simulink model "TASK8_trajectory_tracking"  (R2023b)
settings: Solver=VariableStepAuto  StartTime=0.0  StopTime=80  MaxStep=0.01  RelTol=1e-3  EnableMultiTasking=on
values from neighbouring files (symbols this model uses):
  b = 0.2    [TASK0_main_code.m]
  g = 9.81    [TASK0_main_code.m]
  J_s = 1/3*m*l^2    (= 4.99725166667)    [TASK0_main_code.m]
  K = place(A_lin, B_lin, p)    [TASK0_main_code.m]
  K1 = place(A_lin, B_lin, p1)    [TASK0_main_code.m]
  K2 = place(A_lin, B_lin, p2)    [TASK0_main_code.m]
  K3 = place(A_lin, B_lin, p3)    [TASK0_main_code.m]
  l = 3.11    [TASK0_main_code.m]
  m = 1.55    [TASK0_main_code.m]
  M = 7.87    [TASK0_main_code.m]
  N = [0; 0; 1; 0]    [TASK0_main_code.m]
libraries: dspinverses x4
settings Model: Creator=iklod_000  LastModifiedBy=piri
settings SolverCC: AlgebraicLoopSolver=TrustRegion
settings DataIOCC: ReturnWorkspaceOutputs=off
settings OptimizationCC: LifeSpan=inf
settings DebuggingCC: UnconnectedInputMsg=warning  UnconnectedOutputMsg=warning  UnconnectedLineMsg=warning  SFUnexpectedBacktrackingDiag=warning  SFNoUnconditionalDefaultTransitionDiag=warning  ArithmeticOperatorsInVariantConditions=warning
settings ModelReferenceCC: EnableRefExpFcnMdlSchedulingChecks=on
settings SFSimCC: SimUseLocalCustomCode=off  CustomCodeUndefinedFunction=UseInterfaceOnly
settings RTWCC: RTWUseLocalCustomCode=off
settings CodeAppCC: StateflowObjectComments=on
settings GRTTargetCC: TargetLangStandard=C89/C90 (ANSI)
settings ConfigComp: CovMetricSettings=dw  CovSaveCumulativeToWorkspaceVar=on  CovSaveSingleToWorkspaceVar=on  CovExternalEMLEnable=off

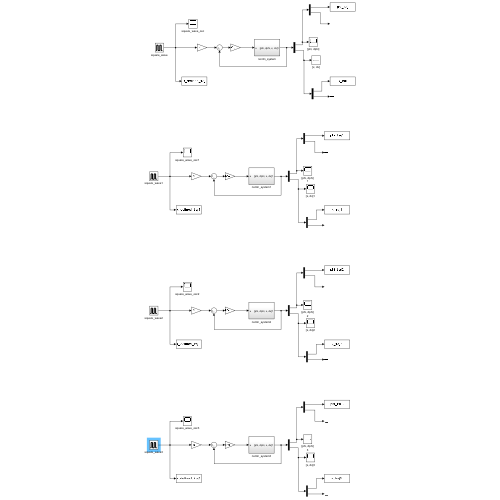
[thumbnail: Simulink's stored preview of the top-level diagram]
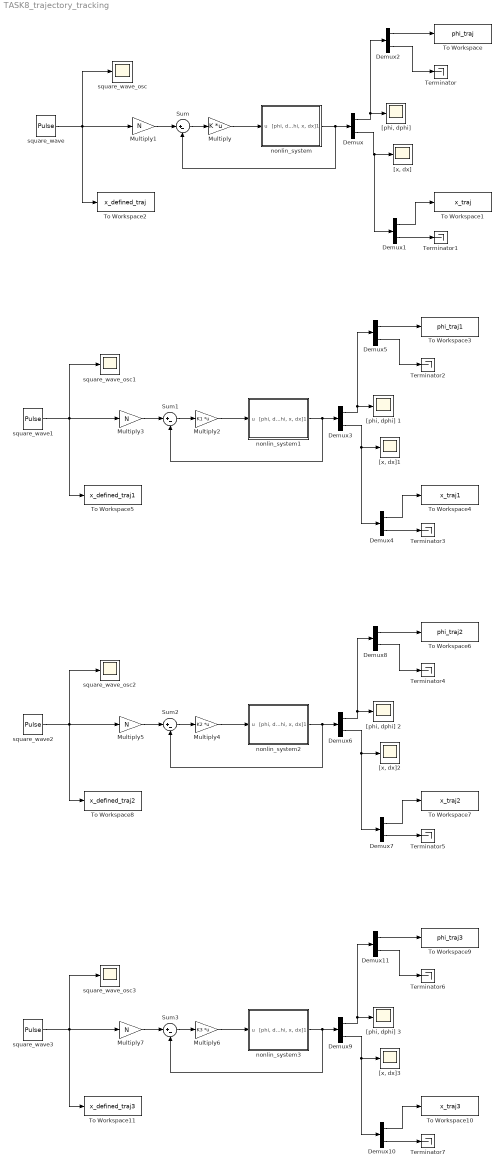
== system TASK8_trajectory_tracking ==
  Demux{,1..11} (12 alike) : Demux  Outputs=2
  Multiply : Gain  Gain=K  Multiplication=Matrix(K*u)
  Multiply{1,3,5,7} (4 alike) : Gain  Gain=N
  Multiply2 : Gain  Gain=K1  Multiplication=Matrix(K*u)
  Multiply4 : Gain  Gain=K2  Multiplication=Matrix(K*u)
  Multiply6 : Gain  Gain=K3  Multiplication=Matrix(K*u)
  Sum{,1..3} (4 alike) : Sum  Inputs=|+-
  Terminator{,1..7} (8 alike) : Terminator
  To Workspace : ToWorkspace  VariableName=phi_traj  SaveFormat=Timeseries  SampleTime=-1
  To Workspace1 : ToWorkspace  VariableName=x_traj  SaveFormat=Timeseries  SampleTime=-1
  To Workspace10 : ToWorkspace  VariableName=x_traj3  SaveFormat=Timeseries  SampleTime=-1
  To Workspace11 : ToWorkspace  VariableName=x_defined_traj3  SaveFormat=Timeseries  SampleTime=-1
  To Workspace2 : ToWorkspace  VariableName=x_defined_traj  SaveFormat=Timeseries  SampleTime=-1
  To Workspace3 : ToWorkspace  VariableName=phi_traj1  SaveFormat=Timeseries  SampleTime=-1
  To Workspace4 : ToWorkspace  VariableName=x_traj1  SaveFormat=Timeseries  SampleTime=-1
  To Workspace5 : ToWorkspace  VariableName=x_defined_traj1  SaveFormat=Timeseries  SampleTime=-1
  To Workspace6 : ToWorkspace  VariableName=phi_traj2  SaveFormat=Timeseries  SampleTime=-1
  To Workspace7 : ToWorkspace  VariableName=x_traj2  SaveFormat=Timeseries  SampleTime=-1
  To Workspace8 : ToWorkspace  VariableName=x_defined_traj2  SaveFormat=Timeseries  SampleTime=-1
  To Workspace9 : ToWorkspace  VariableName=phi_traj3  SaveFormat=Timeseries  SampleTime=-1
  [phi, dphi] {,1..3} (4 alike) : Scope
  [x, dx]{,1..3} (4 alike) : Scope
  nonlin_system : Subsystem
  nonlin_system1 : Subsystem
  nonlin_system2 : Subsystem
  nonlin_system3 : Subsystem
  square_wave{,1..3} (4 alike) : DiscretePulseGenerator  PulseType=Time based  Period=30  PulseWidth=50  PhaseDelay=15
  square_wave_osc{,1..3} (4 alike) : Scope
  wires:
  nonlin_system/1("[phi, dphi, x, dx]1") -> Sum/2, Demux/1
  Demux/1 -> Demux2/1, "[phi, dphi] "/1
  Demux/2 -> Demux1/1, "[x, dx]"/1
  Demux1/2 -> Terminator1/1
  Demux1/1 -> To Workspace1/1
  Demux2/1 -> To Workspace/1
  Demux2/2 -> Terminator/1
  Multiply/1 -> nonlin_system/1(u)
  Sum/1 -> Multiply/1
  Multiply1/1 -> Sum/1
  square_wave/1 -> square_wave_osc/1, To Workspace2/1, Multiply1/1
  Multiply3/1 -> Sum1/1
  Multiply2/1 -> nonlin_system1/1(u)
  square_wave1/1 -> square_wave_osc1/1, To Workspace5/1, Multiply3/1
  Demux3/1 -> Demux5/1, "[phi, dphi] 1"/1
  Demux5/1 -> To Workspace3/1
  Demux5/2 -> Terminator2/1
  Demux4/2 -> Terminator3/1
  nonlin_system1/1("[phi, dphi, x, dx]1") -> Sum1/2, Demux3/1
  Demux4/1 -> To Workspace4/1
  Demux3/2 -> Demux4/1, "[x, dx]1"/1
  Sum1/1 -> Multiply2/1
  Demux7/1 -> To Workspace7/1
  Demux6/2 -> Demux7/1, "[x, dx]2"/1
  Sum2/1 -> Multiply4/1
  Multiply4/1 -> nonlin_system2/1(u)
  Multiply5/1 -> Sum2/1
  square_wave2/1 -> square_wave_osc2/1, To Workspace8/1, Multiply5/1
  nonlin_system2/1("[phi, dphi, x, dx]1") -> Sum2/2, Demux6/1
  Demux8/2 -> Terminator4/1
  Demux8/1 -> To Workspace6/1
  Demux7/2 -> Terminator5/1
  Demux6/1 -> Demux8/1, "[phi, dphi] 2"/1
  Demux10/1 -> To Workspace10/1
  Demux9/2 -> Demux10/1, "[x, dx]3"/1
  Sum3/1 -> Multiply6/1
  Multiply6/1 -> nonlin_system3/1(u)
  Multiply7/1 -> Sum3/1
  square_wave3/1 -> square_wave_osc3/1, To Workspace11/1, Multiply7/1
  nonlin_system3/1("[phi, dphi, x, dx]1") -> Sum3/2, Demux9/1
  Demux11/2 -> Terminator6/1
  Demux11/1 -> To Workspace9/1
  Demux10/2 -> Terminator7/1
  Demux9/1 -> Demux11/1, "[phi, dphi] 3"/1

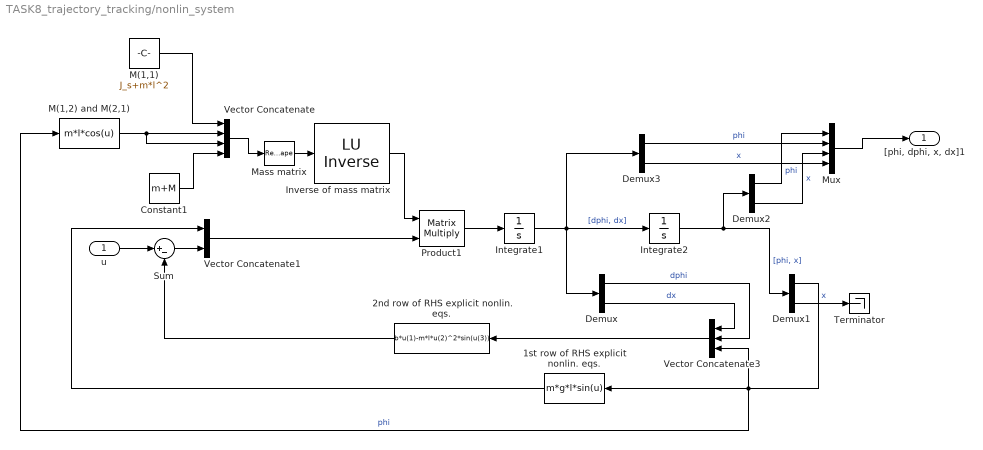
== system TASK8_trajectory_tracking/nonlin_system ==
  u : Inport
  1st row of RHS explicit nonlin. eqs. : Fcn  Expr=m*g*l*sin(u)
  2nd row of RHS explicit nonlin. eqs. : Fcn  Expr=b*u(1)-m*l*u(2)^2*sin(u(3))
  Constant1 : Constant  Value=m+M
  Demux{,1..3} (4 alike) : Demux  Outputs=2
  Integrate1 : Integrator  InitialCondition=[0; 0]
  Integrate2 : Integrator  InitialCondition=[0; 0]
  Inverse of mass matrix : dspinverses/ LU Inverse
  M(1,1) : Constant  Value=J_s+m*l^2
  M(1,2) and M(2,1) : Fcn  Expr=m*l*cos(u)
  Mass matrix : Reshape  OutputDimensionality=Customize  OutputDimensions=[2,2]
  Mux : Mux
  Product1 : Product  Multiplication=Matrix(*)
  Sum : Sum  Inputs=|+-
  Terminator : Terminator
  Vector Concatenate : Concatenate  NumInputs=4
  Vector Concatenate1 : Concatenate
  Vector Concatenate3 : Concatenate  NumInputs=3
  "[phi, dphi, x, dx]1" : Outport
  wires:
  Mass matrix/1 -> Inverse of mass matrix/1
  u/1 -> Sum/1
  Constant1/1 -> Vector Concatenate/4
  Inverse of mass matrix/1 -> Product1/1
  Vector Concatenate3/1 -> 2nd row of RHS explicit nonlin. eqs./1
  Vector Concatenate1/1 -> Product1/2
  1st row of RHS explicit nonlin. eqs./1 -> Vector Concatenate1/1
  Sum/1 -> Vector Concatenate1/2
  2nd row of RHS explicit nonlin. eqs./1 -> Sum/2
  Vector Concatenate/1 -> Mass matrix/1
  M(1,1)/1 -> Vector Concatenate/1
  M(1,2) and M(2,1)/1 -> Vector Concatenate/3, Vector Concatenate/2
  Product1/1 -> Integrate1/1
  Integrate1/1 -> Demux3/1, Demux/1, Integrate2/1  "[dphi, dx]"
  Integrate2/1 -> Demux2/1, Demux1/1  "[phi, x]"
  Demux/2 -> Vector Concatenate3/1  "dx"
  Demux/1 -> Vector Concatenate3/2  "dphi"
  Demux1/1 -> 1st row of RHS explicit nonlin. eqs./1, M(1,2) and M(2,1)/1, Vector Concatenate3/3  "phi"
  Demux2/1 -> Mux/1  "phi"
  Mux/1 -> "[phi, dphi, x, dx]1"/1
  Demux3/1 -> Mux/2  "phi"
  Demux2/2 -> Mux/3  "x"
  Demux3/2 -> Mux/4  "x"
  Demux1/2 -> Terminator/1  "x"

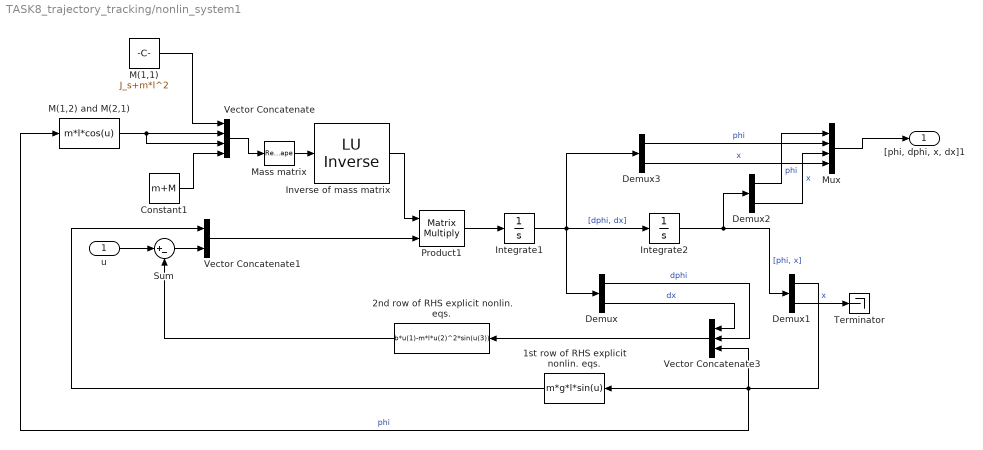
== system TASK8_trajectory_tracking/nonlin_system1 ==
  u : Inport
  1st row of RHS explicit nonlin. eqs. : Fcn  Expr=m*g*l*sin(u)
  2nd row of RHS explicit nonlin. eqs. : Fcn  Expr=b*u(1)-m*l*u(2)^2*sin(u(3))
  Constant1 : Constant  Value=m+M
  Demux{,1..3} (4 alike) : Demux  Outputs=2
  Integrate1 : Integrator  InitialCondition=[0; 0]
  Integrate2 : Integrator  InitialCondition=[0; 0]
  Inverse of mass matrix : dspinverses/ LU Inverse
  M(1,1) : Constant  Value=J_s+m*l^2
  M(1,2) and M(2,1) : Fcn  Expr=m*l*cos(u)
  Mass matrix : Reshape  OutputDimensionality=Customize  OutputDimensions=[2,2]
  Mux : Mux
  Product1 : Product  Multiplication=Matrix(*)
  Sum : Sum  Inputs=|+-
  Terminator : Terminator
  Vector Concatenate : Concatenate  NumInputs=4
  Vector Concatenate1 : Concatenate
  Vector Concatenate3 : Concatenate  NumInputs=3
  "[phi, dphi, x, dx]1" : Outport
  wires:
  Mass matrix/1 -> Inverse of mass matrix/1
  u/1 -> Sum/1
  Constant1/1 -> Vector Concatenate/4
  Inverse of mass matrix/1 -> Product1/1
  Vector Concatenate3/1 -> 2nd row of RHS explicit nonlin. eqs./1
  Vector Concatenate1/1 -> Product1/2
  1st row of RHS explicit nonlin. eqs./1 -> Vector Concatenate1/1
  Sum/1 -> Vector Concatenate1/2
  2nd row of RHS explicit nonlin. eqs./1 -> Sum/2
  Vector Concatenate/1 -> Mass matrix/1
  M(1,1)/1 -> Vector Concatenate/1
  M(1,2) and M(2,1)/1 -> Vector Concatenate/3, Vector Concatenate/2
  Product1/1 -> Integrate1/1
  Integrate1/1 -> Demux3/1, Demux/1, Integrate2/1  "[dphi, dx]"
  Integrate2/1 -> Demux2/1, Demux1/1  "[phi, x]"
  Demux/2 -> Vector Concatenate3/1  "dx"
  Demux/1 -> Vector Concatenate3/2  "dphi"
  Demux1/1 -> 1st row of RHS explicit nonlin. eqs./1, M(1,2) and M(2,1)/1, Vector Concatenate3/3  "phi"
  Demux2/1 -> Mux/1  "phi"
  Mux/1 -> "[phi, dphi, x, dx]1"/1
  Demux3/1 -> Mux/2  "phi"
  Demux2/2 -> Mux/3  "x"
  Demux3/2 -> Mux/4  "x"
  Demux1/2 -> Terminator/1  "x"

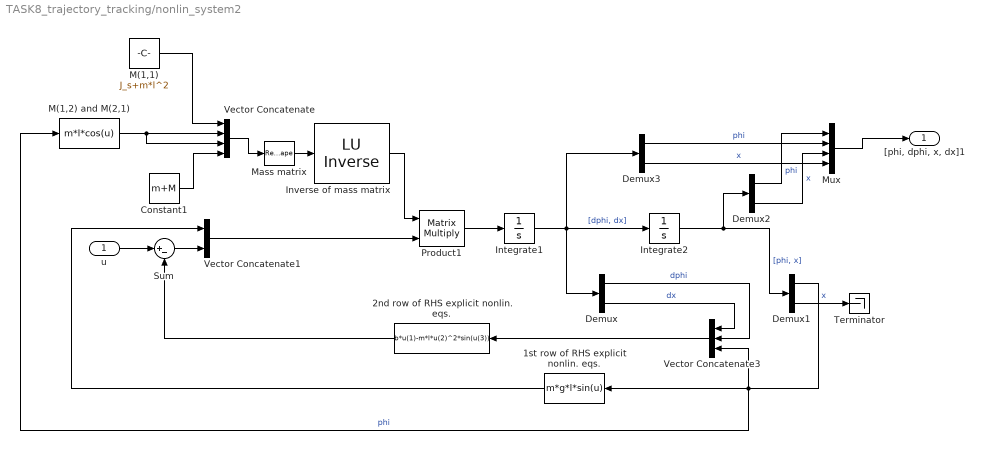
== system TASK8_trajectory_tracking/nonlin_system2 ==
  u : Inport
  1st row of RHS explicit nonlin. eqs. : Fcn  Expr=m*g*l*sin(u)
  2nd row of RHS explicit nonlin. eqs. : Fcn  Expr=b*u(1)-m*l*u(2)^2*sin(u(3))
  Constant1 : Constant  Value=m+M
  Demux{,1..3} (4 alike) : Demux  Outputs=2
  Integrate1 : Integrator  InitialCondition=[0; 0]
  Integrate2 : Integrator  InitialCondition=[0; 0]
  Inverse of mass matrix : dspinverses/ LU Inverse
  M(1,1) : Constant  Value=J_s+m*l^2
  M(1,2) and M(2,1) : Fcn  Expr=m*l*cos(u)
  Mass matrix : Reshape  OutputDimensionality=Customize  OutputDimensions=[2,2]
  Mux : Mux
  Product1 : Product  Multiplication=Matrix(*)
  Sum : Sum  Inputs=|+-
  Terminator : Terminator
  Vector Concatenate : Concatenate  NumInputs=4
  Vector Concatenate1 : Concatenate
  Vector Concatenate3 : Concatenate  NumInputs=3
  "[phi, dphi, x, dx]1" : Outport
  wires:
  Mass matrix/1 -> Inverse of mass matrix/1
  u/1 -> Sum/1
  Constant1/1 -> Vector Concatenate/4
  Inverse of mass matrix/1 -> Product1/1
  Vector Concatenate3/1 -> 2nd row of RHS explicit nonlin. eqs./1
  Vector Concatenate1/1 -> Product1/2
  1st row of RHS explicit nonlin. eqs./1 -> Vector Concatenate1/1
  Sum/1 -> Vector Concatenate1/2
  2nd row of RHS explicit nonlin. eqs./1 -> Sum/2
  Vector Concatenate/1 -> Mass matrix/1
  M(1,1)/1 -> Vector Concatenate/1
  M(1,2) and M(2,1)/1 -> Vector Concatenate/3, Vector Concatenate/2
  Product1/1 -> Integrate1/1
  Integrate1/1 -> Demux3/1, Demux/1, Integrate2/1  "[dphi, dx]"
  Integrate2/1 -> Demux2/1, Demux1/1  "[phi, x]"
  Demux/2 -> Vector Concatenate3/1  "dx"
  Demux/1 -> Vector Concatenate3/2  "dphi"
  Demux1/1 -> 1st row of RHS explicit nonlin. eqs./1, M(1,2) and M(2,1)/1, Vector Concatenate3/3  "phi"
  Demux2/1 -> Mux/1  "phi"
  Mux/1 -> "[phi, dphi, x, dx]1"/1
  Demux3/1 -> Mux/2  "phi"
  Demux2/2 -> Mux/3  "x"
  Demux3/2 -> Mux/4  "x"
  Demux1/2 -> Terminator/1  "x"

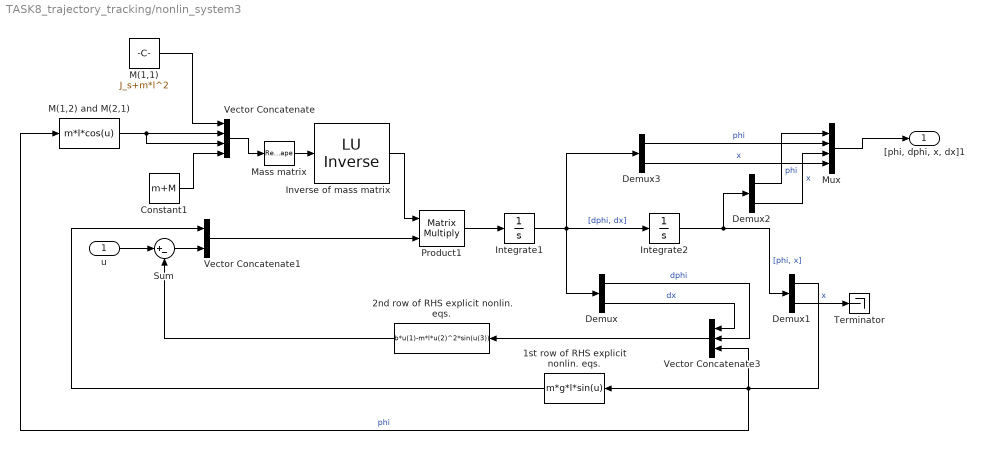
== system TASK8_trajectory_tracking/nonlin_system3 ==
  u : Inport
  1st row of RHS explicit nonlin. eqs. : Fcn  Expr=m*g*l*sin(u)
  2nd row of RHS explicit nonlin. eqs. : Fcn  Expr=b*u(1)-m*l*u(2)^2*sin(u(3))
  Constant1 : Constant  Value=m+M
  Demux{,1..3} (4 alike) : Demux  Outputs=2
  Integrate1 : Integrator  InitialCondition=[0; 0]
  Integrate2 : Integrator  InitialCondition=[0; 0]
  Inverse of mass matrix : dspinverses/ LU Inverse
  M(1,1) : Constant  Value=J_s+m*l^2
  M(1,2) and M(2,1) : Fcn  Expr=m*l*cos(u)
  Mass matrix : Reshape  OutputDimensionality=Customize  OutputDimensions=[2,2]
  Mux : Mux
  Product1 : Product  Multiplication=Matrix(*)
  Sum : Sum  Inputs=|+-
  Terminator : Terminator
  Vector Concatenate : Concatenate  NumInputs=4
  Vector Concatenate1 : Concatenate
  Vector Concatenate3 : Concatenate  NumInputs=3
  "[phi, dphi, x, dx]1" : Outport
  wires:
  Mass matrix/1 -> Inverse of mass matrix/1
  u/1 -> Sum/1
  Constant1/1 -> Vector Concatenate/4
  Inverse of mass matrix/1 -> Product1/1
  Vector Concatenate3/1 -> 2nd row of RHS explicit nonlin. eqs./1
  Vector Concatenate1/1 -> Product1/2
  1st row of RHS explicit nonlin. eqs./1 -> Vector Concatenate1/1
  Sum/1 -> Vector Concatenate1/2
  2nd row of RHS explicit nonlin. eqs./1 -> Sum/2
  Vector Concatenate/1 -> Mass matrix/1
  M(1,1)/1 -> Vector Concatenate/1
  M(1,2) and M(2,1)/1 -> Vector Concatenate/3, Vector Concatenate/2
  Product1/1 -> Integrate1/1
  Integrate1/1 -> Demux3/1, Demux/1, Integrate2/1  "[dphi, dx]"
  Integrate2/1 -> Demux2/1, Demux1/1  "[phi, x]"
  Demux/2 -> Vector Concatenate3/1  "dx"
  Demux/1 -> Vector Concatenate3/2  "dphi"
  Demux1/1 -> 1st row of RHS explicit nonlin. eqs./1, M(1,2) and M(2,1)/1, Vector Concatenate3/3  "phi"
  Demux2/1 -> Mux/1  "phi"
  Mux/1 -> "[phi, dphi, x, dx]1"/1
  Demux3/1 -> Mux/2  "phi"
  Demux2/2 -> Mux/3  "x"
  Demux3/2 -> Mux/4  "x"
  Demux1/2 -> Terminator/1  "x"
